simulink library "StateEstimation_lib"  (R2016b)
settings: Solver=VariableStepAuto  StartTime=0.0  StopTime=10.0  RelTol=1e-3
values from neighbouring files (symbols this model uses):
  accel_bias_init = zeros(3,1)    [Copy_of_StateEstimator_RIEKF.m]    (also in Quaternion_EKF.m; RightInvariant_EKF.m; StateEstimator_EKF.m; StateEstimator_RIEKF.m)
  accel_bias_noise_std = 0.1*ones(3,1)    [Copy_of_StateEstimator_RIEKF.m]    (also in Quaternion_EKF.m; RightInvariant_EKF.m; StateEstimator_EKF.m; StateEstimator_RIEKF.m)
  accel_noise_std = 0.1*ones(3,1)    [Copy_of_StateEstimator_RIEKF.m]    (also in Quaternion_EKF.m; RightInvariant_EKF.m; StateEstimator_EKF.m; StateEstimator_RIEKF.m)
  gyro_bias_init = zeros(3,1)    [Copy_of_StateEstimator_RIEKF.m]    (also in Quaternion_EKF.m; RightInvariant_EKF.m; StateEstimator_EKF.m; StateEstimator_RIEKF.m)
  gyro_bias_noise_std = 0.1*ones(3,1)    [Copy_of_StateEstimator_RIEKF.m]    (also in Quaternion_EKF.m; RightInvariant_EKF.m; StateEstimator_EKF.m; StateEstimator_RIEKF.m)
  gyro_noise_std = 0.1*ones(3,1)    [Copy_of_StateEstimator_RIEKF.m]    (also in Quaternion_EKF.m; RightInvariant_EKF.m; StateEstimator_EKF.m; StateEstimator_RIEKF.m)
undefined symbols (not defined in the file or in its folder): cassieParameters, CassieParameters, EKF_SampleTime, q_init, v_init
libraries: xpcutilitieslib x41, xpcrtudplib x41, dspfdesign x10, simulink x6, slrtlib x5
(part 4 of 4)

== matlab function StateEstimation_lib/Quaternion-based EKF/Reconstruct State/Construct_State ==
  data: q output; dq output; q input; dq input; w input; contact input; mu input; ekf_enabled input; velocity output; velocity_kinematic output; filter_selector output
function [q, dq, velocity, velocity_kinematic, filter_selector] = Construct_State(q, dq, w, contact, mu, ekf_enabled)
% Construct state vector and body velocity estimate using raw data and ekf
%   
%   Inputs:
%       q           - state position vector
%       dq          - state velocity vector
%       w           - angular velocity, {I}_\omega_{WI}
%       contact     - contact indicator
%       mu          - EKF state estimate
%       ekf_enabled - EKF enable flag
%
%   Outputs:
%       q                   - 
%       dq                  - 
%       velocity            - EKF body velocity, {W}_v_{WB} 
%       velocity_kinematic  - Kinematic body velocity, {B}_v_{WB} 
%       filter_selector     - used to select low pass filter type
%
%
%   Author: Ross Hartley
%   Date:   11/07/2017

%% Settings
use_ekf_position = true;
use_ekf_orientation = false;
use_ekf_velocity = false;

%% Compute kinematic velocity
e = q(7:end);
e_dot = dq(7:end);

if contact(1) == 1
    pL = p_VectorNav_to_LeftToeBottom(e); % {I}_p_{IL}
    J_pL = J_VectorNav_to_LeftToeBottom(e);
    velocity_kinematic = -J_pL(1:3,:)*e_dot - Angles.skew(w)*pL(1:3,:); % {I}_v_{WI}
elseif contact(2) == 1
    pR = p_VectorNav_to_RightToeBottom(e); % {I}_p_{IR}
    J_pR = J_VectorNav_to_RightToeBottom(e);
    velocity_kinematic = -J_pR(1:3,:)*e_dot - Angles.skew(w)*pR(1:3,:); % {I}_v_{WI}
else
    velocity_kinematic = zeros(3,1);
end

%% Reconstruct State
Rbi = R_VectorNav_to_Pelvis(e)';    % R_{BI}

% Position
if use_ekf_position && ekf_enabled
    Rwi = Angles.Quaternion_to_Rotation(mu(7:10))';
    % {W}_p_{WB} =  {W}_p_{WI} +  {W}_p_{IB}
    q(1:3) = mu(1:3) + Rwi * p_VectorNav_to_Pelvis(e); 
end
 
% Orientation
if use_ekf_orientation && ekf_enabled
    Rwi = Angles.Quaternion_to_Rotation(mu(7:10))';
    Rwb = Rwi * Rbi';
    q(4:6) = Angles.Rotation_to_Euler( Rwb );
end

% Velocity
if use_ekf_velocity && ekf_enabled
    Rwi = Angles.Quaternion_to_Rotation(mu(7:10))';
    Rwb = Rwi * Rbi';
    % {W}_v_{WB} =  {W}_v_{WI} + R_{WI} * skew({I}_w_{WI}) * {I}_p_{IB}
    dq(1:3) = mu(4:6) + Rwi * Angles.skew(w) * p_VectorNav_to_Pelvis(e); 
    % {B}_v_{WB} = R_{BW} * {W}_v_{WB}
    velocity = Rwb' * dq(1:3);
    filter_selector = 1;
else
    Rwb = Angles.Euler_to_Rotation(q(4:6));
    Rwi = Rwb * Rbi;
    % {W}_v_{WB} =  R_{WI} * {I}_v_{WI} + R_{WI} * skew({I}_w_{WI}) * {I}_p_{IB}
    dq(1:3) = Rwi * velocity_kinematic + Rwi * Angles.skew(w) * p_VectorNav_to_Pelvis(e); 
    % {B}_v_{WB} = R_{BW} * {W}_v_{WB}
    velocity = Rwb' * dq(1:3);
    filter_selector = 0;
end



end
